simulink model "Ieee14_CC_2019b"  (R2019b)
settings: Solver=ode1  StartTime=0.0  StopTime=3600  FixedStep=1e-3  MaxStep=1e-4  RelTol=1e-3
model workspace (MAT data in the model file):
  pruebaValor = 0
libraries: powerlib x118, dspnetwork x112, source_mod x14, realtime_pacer_lib x1
(part 3 of 3)

== system Ieee14_CC_2019b/SM 5 ==
  Constant : Constant  Value=0
  Constant1 : Constant
  Constant2 : Constant  Value=2
  Constant3 : Constant  Value=0
  Constant4 : Constant
  Constant5 : Constant  Value=2
  Index Vector{,1..5} (6 alike) : MultiPortSwitch  DataPortOrder=Zero-based contiguous  Inputs=1  zeroidx=on
  Three-Phase V-I Measurement : powerlib/Measurements/Three-Phase V-I Measurement  VoltageMeasurement=phase-to-ground  SetLabelV=off  LabelV=Vabc  Vpu=on  VpuLL=off  CurrentMeasurement=yes  SetLabelI=off  LabelI=Iabc  Ipu=on  Pbase=100e6  Vbase=69e3  OutputType=Complex  PhasorSimulation=off  PSBequivalent=0
  UDP Send Ia : dspnetwork/UDP Send  remoteURL='10.0.255.255'  remotePort=20052  localURL='255.255.255.255'  localPortSource=Automatically determine  localPort=-1  sampletime=-1  blockPlatform=LINUX  separateLengthPort=0
  UDP Send Ib : dspnetwork/UDP Send  remoteURL='10.0.255.255'  remotePort=20051  localURL='255.255.255.255'  localPortSource=Automatically determine  localPort=-1  sampletime=-1  blockPlatform=LINUX  separateLengthPort=0
  UDP Send Ic : dspnetwork/UDP Send  remoteURL='10.0.255.255'  remotePort=20050  localURL='255.255.255.255'  localPortSource=Automatically determine  localPort=-1  sampletime=-1  blockPlatform=LINUX  separateLengthPort=0
  UDP Send Va : dspnetwork/UDP Send  remoteURL='10.0.255.255'  remotePort=10050  localURL='255.255.255.255'  localPortSource=Automatically determine  localPort=-1  sampletime=-1  blockPlatform=LINUX  separateLengthPort=0
  UDP Send Vb : dspnetwork/UDP Send  remoteURL='10.0.255.255'  remotePort=10051  localURL='255.255.255.255'  localPortSource=Automatically determine  localPort=-1  sampletime=-1  blockPlatform=LINUX  separateLengthPort=0
  UDP Send Vc : dspnetwork/UDP Send  remoteURL='10.0.255.255'  remotePort=10052  localURL='255.255.255.255'  localPortSource=Automatically determine  localPort=-1  sampletime=-1  blockPlatform=LINUX  separateLengthPort=0
  a : PMIOPort  Side=Left
  b : PMIOPort  Port=2  Side=Left
  c : PMIOPort  Port=3  Side=Left
  A : PMIOPort  Port=4  Side=Right
  B : PMIOPort  Port=5  Side=Right
  C : PMIOPort  Port=6  Side=Right
  Vabc : Outport
  Iabc : Outport  Port=2
  wires:
  Index Vector/1 -> UDP Send Va/1
  Constant1/1 -> Index Vector1/1
  Constant/1 -> Index Vector/1
  Index Vector2/1 -> UDP Send Vc/1
  Index Vector1/1 -> UDP Send Vb/1
  Constant2/1 -> Index Vector2/1
  Three-Phase V-I Measurement/1 -> Index Vector2/2, Index Vector/2, Index Vector1/2, Vabc/1
  Index Vector4/1 -> UDP Send Ib/1
  Constant3/1 -> Index Vector3/1
  Index Vector3/1 -> UDP Send Ic/1
  Constant5/1 -> Index Vector5/1
  Constant4/1 -> Index Vector4/1
  Index Vector5/1 -> UDP Send Ia/1
  Three-Phase V-I Measurement/2 -> Iabc/1, Index Vector3/2, Index Vector4/2, Index Vector5/2
  connections:
  b/RConn1 -- Three-Phase V-I Measurement/RConn2
  a/RConn1 -- Three-Phase V-I Measurement/RConn1
  c/RConn1 -- Three-Phase V-I Measurement/RConn3
  A/RConn1 -- Three-Phase V-I Measurement/LConn1
  B/RConn1 -- Three-Phase V-I Measurement/LConn2
  C/RConn1 -- Three-Phase V-I Measurement/LConn3

== system Ieee14_CC_2019b/SM 6 ==
  Constant : Constant  Value=0
  Constant1 : Constant
  Constant2 : Constant  Value=2
  Constant3 : Constant  Value=0
  Constant4 : Constant
  Constant5 : Constant  Value=2
  Index Vector{,1..5} (6 alike) : MultiPortSwitch  DataPortOrder=Zero-based contiguous  Inputs=1  zeroidx=on
  Three-Phase V-I Measurement : powerlib/Measurements/Three-Phase V-I Measurement  VoltageMeasurement=phase-to-ground  SetLabelV=off  LabelV=Vabc  Vpu=on  VpuLL=off  CurrentMeasurement=yes  SetLabelI=off  LabelI=Iabc  Ipu=on  Pbase=100e6  Vbase=69e3  OutputType=Complex  PhasorSimulation=off  PSBequivalent=0
  UDP Send Ia : dspnetwork/UDP Send  remoteURL='10.0.255.255'  remotePort=20062  localURL='255.255.255.255'  localPortSource=Automatically determine  localPort=-1  sampletime=-1  blockPlatform=LINUX  separateLengthPort=0
  UDP Send Ib : dspnetwork/UDP Send  remoteURL='10.0.255.255'  remotePort=20061  localURL='255.255.255.255'  localPortSource=Automatically determine  localPort=-1  sampletime=-1  blockPlatform=LINUX  separateLengthPort=0
  UDP Send Ic : dspnetwork/UDP Send  remoteURL='10.0.255.255'  remotePort=20060  localURL='255.255.255.255'  localPortSource=Automatically determine  localPort=-1  sampletime=-1  blockPlatform=LINUX  separateLengthPort=0
  UDP Send Va : dspnetwork/UDP Send  remoteURL='10.0.255.255'  remotePort=10060  localURL='255.255.255.255'  localPortSource=Automatically determine  localPort=-1  sampletime=-1  blockPlatform=LINUX  separateLengthPort=0
  UDP Send Vb : dspnetwork/UDP Send  remoteURL='10.0.255.255'  remotePort=10061  localURL='255.255.255.255'  localPortSource=Automatically determine  localPort=-1  sampletime=-1  blockPlatform=LINUX  separateLengthPort=0
  UDP Send Vc : dspnetwork/UDP Send  remoteURL='10.0.255.255'  remotePort=10062  localURL='255.255.255.255'  localPortSource=Automatically determine  localPort=-1  sampletime=-1  blockPlatform=LINUX  separateLengthPort=0
  a : PMIOPort  Side=Left
  b : PMIOPort  Port=2  Side=Left
  c : PMIOPort  Port=3  Side=Left
  A : PMIOPort  Port=4  Side=Right
  B : PMIOPort  Port=5  Side=Right
  C : PMIOPort  Port=6  Side=Right
  Vabc : Outport
  Iabc : Outport  Port=2
  wires:
  Index Vector/1 -> UDP Send Va/1
  Constant1/1 -> Index Vector1/1
  Constant/1 -> Index Vector/1
  Index Vector2/1 -> UDP Send Vc/1
  Index Vector1/1 -> UDP Send Vb/1
  Constant2/1 -> Index Vector2/1
  Three-Phase V-I Measurement/1 -> Index Vector2/2, Index Vector/2, Index Vector1/2, Vabc/1
  Index Vector4/1 -> UDP Send Ib/1
  Constant3/1 -> Index Vector3/1
  Index Vector3/1 -> UDP Send Ic/1
  Constant5/1 -> Index Vector5/1
  Constant4/1 -> Index Vector4/1
  Index Vector5/1 -> UDP Send Ia/1
  Three-Phase V-I Measurement/2 -> Iabc/1, Index Vector3/2, Index Vector4/2, Index Vector5/2
  connections:
  b/RConn1 -- Three-Phase V-I Measurement/RConn2
  a/RConn1 -- Three-Phase V-I Measurement/RConn1
  c/RConn1 -- Three-Phase V-I Measurement/RConn3
  A/RConn1 -- Three-Phase V-I Measurement/LConn1
  B/RConn1 -- Three-Phase V-I Measurement/LConn2
  C/RConn1 -- Three-Phase V-I Measurement/LConn3

== system Ieee14_CC_2019b/SM 7 ==
  Constant : Constant  Value=0
  Constant1 : Constant
  Constant2 : Constant  Value=2
  Constant3 : Constant  Value=0
  Constant4 : Constant
  Constant5 : Constant  Value=2
  Index Vector{,1..5} (6 alike) : MultiPortSwitch  DataPortOrder=Zero-based contiguous  Inputs=1  zeroidx=on
  Three-Phase V-I Measurement : powerlib/Measurements/Three-Phase V-I Measurement  VoltageMeasurement=phase-to-ground  SetLabelV=off  LabelV=Vabc  Vpu=on  VpuLL=off  CurrentMeasurement=yes  SetLabelI=off  LabelI=Iabc  Ipu=on  Pbase=100e6  Vbase=69e3  OutputType=Complex  PhasorSimulation=off  PSBequivalent=0
  UDP Send Ia : dspnetwork/UDP Send  remoteURL='10.0.255.255'  remotePort=20072  localURL='255.255.255.255'  localPortSource=Automatically determine  localPort=-1  sampletime=-1  blockPlatform=LINUX  separateLengthPort=0
  UDP Send Ib : dspnetwork/UDP Send  remoteURL='10.0.255.255'  remotePort=20071  localURL='255.255.255.255'  localPortSource=Automatically determine  localPort=-1  sampletime=-1  blockPlatform=LINUX  separateLengthPort=0
  UDP Send Ic : dspnetwork/UDP Send  remoteURL='10.0.255.255'  remotePort=20070  localURL='255.255.255.255'  localPortSource=Automatically determine  localPort=-1  sampletime=-1  blockPlatform=LINUX  separateLengthPort=0
  UDP Send Va : dspnetwork/UDP Send  remoteURL='10.0.255.255'  remotePort=10070  localURL='255.255.255.255'  localPortSource=Automatically determine  localPort=-1  sampletime=-1  blockPlatform=LINUX  separateLengthPort=0
  UDP Send Vb : dspnetwork/UDP Send  remoteURL='10.0.255.255'  remotePort=10071  localURL='255.255.255.255'  localPortSource=Automatically determine  localPort=-1  sampletime=-1  blockPlatform=LINUX  separateLengthPort=0
  UDP Send Vc : dspnetwork/UDP Send  remoteURL='10.0.255.255'  remotePort=10072  localURL='255.255.255.255'  localPortSource=Automatically determine  localPort=-1  sampletime=-1  blockPlatform=LINUX  separateLengthPort=0
  a : PMIOPort  Side=Left
  b : PMIOPort  Port=2  Side=Left
  c : PMIOPort  Port=3  Side=Left
  A : PMIOPort  Port=4  Side=Right
  B : PMIOPort  Port=5  Side=Right
  C : PMIOPort  Port=6  Side=Right
  Vabc : Outport
  Iabc : Outport  Port=2
  wires:
  Index Vector/1 -> UDP Send Va/1
  Constant1/1 -> Index Vector1/1
  Constant/1 -> Index Vector/1
  Index Vector2/1 -> UDP Send Vc/1
  Index Vector1/1 -> UDP Send Vb/1
  Constant2/1 -> Index Vector2/1
  Three-Phase V-I Measurement/1 -> Index Vector2/2, Index Vector/2, Index Vector1/2, Vabc/1
  Index Vector4/1 -> UDP Send Ib/1
  Constant3/1 -> Index Vector3/1
  Index Vector3/1 -> UDP Send Ic/1
  Constant5/1 -> Index Vector5/1
  Constant4/1 -> Index Vector4/1
  Index Vector5/1 -> UDP Send Ia/1
  Three-Phase V-I Measurement/2 -> Iabc/1, Index Vector3/2, Index Vector4/2, Index Vector5/2
  connections:
  b/RConn1 -- Three-Phase V-I Measurement/RConn2
  a/RConn1 -- Three-Phase V-I Measurement/RConn1
  c/RConn1 -- Three-Phase V-I Measurement/RConn3
  A/RConn1 -- Three-Phase V-I Measurement/LConn1
  B/RConn1 -- Three-Phase V-I Measurement/LConn2
  C/RConn1 -- Three-Phase V-I Measurement/LConn3

== system Ieee14_CC_2019b/SM 8 ==
  Constant : Constant  Value=0
  Constant1 : Constant
  Constant2 : Constant  Value=2
  Constant3 : Constant  Value=0
  Constant4 : Constant
  Constant5 : Constant  Value=2
  Index Vector{,1..5} (6 alike) : MultiPortSwitch  DataPortOrder=Zero-based contiguous  Inputs=1  zeroidx=on
  Three-Phase V-I Measurement : powerlib/Measurements/Three-Phase V-I Measurement  VoltageMeasurement=phase-to-ground  SetLabelV=off  LabelV=Vabc  Vpu=on  VpuLL=off  CurrentMeasurement=yes  SetLabelI=off  LabelI=Iabc  Ipu=on  Pbase=100e6  Vbase=69e3  OutputType=Complex  PhasorSimulation=off  PSBequivalent=0
  UDP Send Ia : dspnetwork/UDP Send  remoteURL='10.0.255.255'  remotePort=20082  localURL='255.255.255.255'  localPortSource=Automatically determine  localPort=-1  sampletime=-1  blockPlatform=LINUX  separateLengthPort=0
  UDP Send Ib : dspnetwork/UDP Send  remoteURL='10.0.255.255'  remotePort=20081  localURL='255.255.255.255'  localPortSource=Automatically determine  localPort=-1  sampletime=-1  blockPlatform=LINUX  separateLengthPort=0
  UDP Send Ic : dspnetwork/UDP Send  remoteURL='10.0.255.255'  remotePort=20080  localURL='255.255.255.255'  localPortSource=Automatically determine  localPort=-1  sampletime=-1  blockPlatform=LINUX  separateLengthPort=0
  UDP Send Va : dspnetwork/UDP Send  remoteURL='10.0.255.255'  remotePort=10080  localURL='255.255.255.255'  localPortSource=Automatically determine  localPort=-1  sampletime=-1  blockPlatform=LINUX  separateLengthPort=0
  UDP Send Vb : dspnetwork/UDP Send  remoteURL='10.0.255.255'  remotePort=10081  localURL='255.255.255.255'  localPortSource=Automatically determine  localPort=-1  sampletime=-1  blockPlatform=LINUX  separateLengthPort=0
  UDP Send Vc : dspnetwork/UDP Send  remoteURL='10.0.255.255'  remotePort=10082  localURL='255.255.255.255'  localPortSource=Automatically determine  localPort=-1  sampletime=-1  blockPlatform=LINUX  separateLengthPort=0
  a : PMIOPort  Side=Left
  b : PMIOPort  Port=2  Side=Left
  c : PMIOPort  Port=3  Side=Left
  A : PMIOPort  Port=4  Side=Right
  B : PMIOPort  Port=5  Side=Right
  C : PMIOPort  Port=6  Side=Right
  Vabc : Outport
  Iabc : Outport  Port=2
  wires:
  Index Vector/1 -> UDP Send Va/1
  Constant1/1 -> Index Vector1/1
  Constant/1 -> Index Vector/1
  Index Vector2/1 -> UDP Send Vc/1
  Index Vector1/1 -> UDP Send Vb/1
  Constant2/1 -> Index Vector2/1
  Three-Phase V-I Measurement/1 -> Index Vector2/2, Index Vector/2, Index Vector1/2, Vabc/1
  Index Vector4/1 -> UDP Send Ib/1
  Constant3/1 -> Index Vector3/1
  Index Vector3/1 -> UDP Send Ic/1
  Constant5/1 -> Index Vector5/1
  Constant4/1 -> Index Vector4/1
  Index Vector5/1 -> UDP Send Ia/1
  Three-Phase V-I Measurement/2 -> Iabc/1, Index Vector3/2, Index Vector4/2, Index Vector5/2
  connections:
  b/RConn1 -- Three-Phase V-I Measurement/RConn2
  a/RConn1 -- Three-Phase V-I Measurement/RConn1
  c/RConn1 -- Three-Phase V-I Measurement/RConn3
  A/RConn1 -- Three-Phase V-I Measurement/LConn1
  B/RConn1 -- Three-Phase V-I Measurement/LConn2
  C/RConn1 -- Three-Phase V-I Measurement/LConn3

== system Ieee14_CC_2019b/SM 9 ==
  Constant : Constant  Value=0
  Constant1 : Constant
  Constant2 : Constant  Value=2
  Constant3 : Constant  Value=0
  Constant4 : Constant
  Constant5 : Constant  Value=2
  Index Vector{,1..5} (6 alike) : MultiPortSwitch  DataPortOrder=Zero-based contiguous  Inputs=1  zeroidx=on
  Three-Phase V-I Measurement : powerlib/Measurements/Three-Phase V-I Measurement  VoltageMeasurement=phase-to-ground  SetLabelV=off  LabelV=Vabc  Vpu=on  VpuLL=off  CurrentMeasurement=yes  SetLabelI=off  LabelI=Iabc  Ipu=on  Pbase=100e6  Vbase=69e3  OutputType=Complex  PhasorSimulation=off  PSBequivalent=0
  UDP Send Ia : dspnetwork/UDP Send  remoteURL='10.0.255.255'  remotePort=20092  localURL='255.255.255.255'  localPortSource=Automatically determine  localPort=-1  sampletime=-1  blockPlatform=LINUX  separateLengthPort=0
  UDP Send Ib : dspnetwork/UDP Send  remoteURL='10.0.255.255'  remotePort=20091  localURL='255.255.255.255'  localPortSource=Automatically determine  localPort=-1  sampletime=-1  blockPlatform=LINUX  separateLengthPort=0
  UDP Send Ic : dspnetwork/UDP Send  remoteURL='10.0.255.255'  remotePort=20090  localURL='255.255.255.255'  localPortSource=Automatically determine  localPort=-1  sampletime=-1  blockPlatform=LINUX  separateLengthPort=0
  UDP Send Va : dspnetwork/UDP Send  remoteURL='10.0.255.255'  remotePort=10090  localURL='255.255.255.255'  localPortSource=Automatically determine  localPort=-1  sampletime=-1  blockPlatform=LINUX  separateLengthPort=0
  UDP Send Vb : dspnetwork/UDP Send  remoteURL='10.0.255.255'  remotePort=10091  localURL='255.255.255.255'  localPortSource=Automatically determine  localPort=-1  sampletime=-1  blockPlatform=LINUX  separateLengthPort=0
  UDP Send Vc : dspnetwork/UDP Send  remoteURL='10.0.255.255'  remotePort=10092  localURL='255.255.255.255'  localPortSource=Automatically determine  localPort=-1  sampletime=-1  blockPlatform=LINUX  separateLengthPort=0
  a : PMIOPort  Side=Left
  b : PMIOPort  Port=2  Side=Left
  c : PMIOPort  Port=3  Side=Left
  A : PMIOPort  Port=4  Side=Right
  B : PMIOPort  Port=5  Side=Right
  C : PMIOPort  Port=6  Side=Right
  Vabc : Outport
  Iabc : Outport  Port=2
  wires:
  Index Vector/1 -> UDP Send Va/1
  Constant1/1 -> Index Vector1/1
  Constant/1 -> Index Vector/1
  Index Vector2/1 -> UDP Send Vc/1
  Index Vector1/1 -> UDP Send Vb/1
  Constant2/1 -> Index Vector2/1
  Three-Phase V-I Measurement/1 -> Index Vector2/2, Index Vector/2, Index Vector1/2, Vabc/1
  Index Vector4/1 -> UDP Send Ib/1
  Constant3/1 -> Index Vector3/1
  Index Vector3/1 -> UDP Send Ic/1
  Constant5/1 -> Index Vector5/1
  Constant4/1 -> Index Vector4/1
  Index Vector5/1 -> UDP Send Ia/1
  Three-Phase V-I Measurement/2 -> Iabc/1, Index Vector3/2, Index Vector4/2, Index Vector5/2
  connections:
  b/RConn1 -- Three-Phase V-I Measurement/RConn2
  a/RConn1 -- Three-Phase V-I Measurement/RConn1
  c/RConn1 -- Three-Phase V-I Measurement/RConn3
  A/RConn1 -- Three-Phase V-I Measurement/LConn1
  B/RConn1 -- Three-Phase V-I Measurement/LConn2
  C/RConn1 -- Three-Phase V-I Measurement/LConn3

== matlab function Ieee14_CC_2019b/CC ==
  settings: updateMethod=DISCRETE  sampleTime=10
function fcn()

    %{
    
    Function CC: short circuits.
    
    Details: This function is responsible for causing short circuits throughout the simulation.
    
    Important: In edit Data, you must adjust the time interval for entering this function. If the interval is set to 5 seconds, its behavior is:
    
    T = 5s --> A random fault is activated
    T = 10s --> The fault is deactivated
    T = 15s --> A random fault is activated
    T = 20s --> The fault is deactivated
    ... ... ...
    
    %}

    
    % - - - - - - - - - - - - - - - - - - - - - - - - -
    
    % coders
    coder.extrinsic('mat2str');
    coder.extrinsic('set_param');
    
    % - - - - - - - - - - - - - - - - - - - - - - - - -
    
    % If skip=1, no fault is activated
    skip = 0;
    
    % - - - - - - - - - - - - - - - - - - - - - - - - -
    
    % = = = = = = = = = = = = = = = = = = = = = = = = =
    % = = = = = = = = = = = = = = = = = = = = = = = = =
    % - - - - - - - - Code - - - - - - - - - - - - - 
    % = = = = = = = = = = = = = = = = = = = = = = = = =
    % = = = = = = = = = = = = = = = = = = = = = = = = =
    
    % - - - - - - - - - - - - - - - - - - - - - - - - -
    
    % Activate or skip fault generation
    if skip == 1
        return
    end
    
    % - - - - - - - - - - - - - - - - - - - - - - - - -
    
    % Persisten variables
    
    % attack: if 1, fault is activated (cc)
    persistent fault_active
    if isempty(fault_active)
       fault_active = 0;
       return
    end
    
    % lineCC: line with active fault
    persistent lineCC;
    if isempty(lineCC)
        lineCC = 0;
    end
    
    % - - - - - - - - - - - - - - - - - - - - - - - - -
    
    % Model path
    path = "Ieee14_CC/";
    
    % - - - - - - - - - - - - - - - - - - - - - - - - -
    
    % Restore ataque
    if fault_active == 1
        if lineCC == 0
            line = "L0";
            aux = path + "CC_" + line;
            set_param(aux, 'Value', mat2str(0));
        end
        if lineCC == 1
            line = "L1";
            aux = path + "CC_" + line;
            set_param(aux, 'Value', mat2str(0));
        end
        if lineCC == 2
            line = "L2";
            aux = path + "CC_" + line;
            set_param(aux, 'Value', mat2str(0));
        end
        if lineCC == 3
            line = "L3";
            aux = path + "CC_" + line;
            set_param(aux, 'Value', mat2str(0));
        end
        if lineCC == 4
            line = "L4";
            aux = path + "CC_" + line;
            set_param(aux, 'Value', mat2str(0));
        end
        if lineCC == 5
            line = "L5";
            aux = path + "CC_" + line;
            set_param(aux, 'Value', mat2str(0));
        end
        if lineCC == 6
            line = "L6";
            aux = path + "CC_" + line;
            set_param(aux, 'Value', mat2str(0));
        end
        if lineCC == 7
            line = "L7";
            aux = path + "CC_" + line;
            set_param(aux, 'Value', mat2str(0));
        end
        if lineCC == 8
            line = "L8";
            aux = path + "CC_" + line;
            set_param(aux, 'Value', mat2str(0));
        end
        if lineCC == 9
            line = "L9";
            aux = path + "CC_" + line;
            set_param(aux, 'Value', mat2str(0));
        end
        if lineCC == 10
            line = "L10";
            aux = path + "CC_" + line;
            set_param(aux, 'Value', mat2str(0));
        end
        if lineCC == 11
            line = "L11";
            aux = path + "CC_" + line;
            set_param(aux, 'Value', mat2str(0));
        end
        if lineCC == 12
            line = "L12";
            aux = path + "CC_" + line;
            set_param(aux, 'Value', mat2str(0));
        end
        if lineCC == 13
            line = "L13";
            aux = path + "CC_" + line;
            set_param(aux, 'Value', mat2str(0));
        end
        if lineCC == 14
            line = "L14";
            aux = path + "CC_" + line;
            set_param(aux, 'Value', mat2str(0));
        end
        if lineCC == 15
            line = "L15";
            aux = path + "CC_" + line;
            set_param(aux, 'Value', mat2str(0));
        end
    
        fault_active = 0;
        disp('=============')
        disp('Disconnection CC');
        disp('=============');
        return
    end
    
    % Activate fault

    % Probability of 10% of line failing
    activate = randi(10);
    
    if fault_active == 0 && activate
        % Randomly select line (0-15)
        lineCC = randi(16) - 1;
        disp('=======================');
        disp('=======================');
        disp('LineaCC');
        disp(lineCC);
        disp('=======================');
        disp('=======================');
        if lineCC == 0
            line = "L0";
            aux = path + "CC_" + line;
            set_param(aux, 'Value', mat2str(1));
        end
        if lineCC == 1
            line = "L1";
            aux = path + "CC_" + line;
            set_param(aux, 'Value', mat2str(1));
        end
        if lineCC == 2
            line = "L2";
            aux = path + "CC_" + line;
            set_param(aux, 'Value', mat2str(1));
        end
        if lineCC == 3
            line = "L3";
            aux = path + "CC_" + line;
            set_param(aux, 'Value', mat2str(1));
        end
        if lineCC == 4
            line = "L4";
            aux = path + "CC_" + line;
            set_param(aux, 'Value', mat2str(1));
        end
        if lineCC == 5
            line = "L5";
            aux = path + "CC_" + line;
            set_param(aux, 'Value', mat2str(1));
        end
        if lineCC == 6
            line = "L6";
            aux = path + "CC_" + line;
            set_param(aux, 'Value', mat2str(1));
        end
        if lineCC == 7
            line = "L7";
            aux = path + "CC_" + line;
            set_param(aux, 'Value', mat2str(1));
        end
        if lineCC == 8
            line = "L8";
            aux = path + "CC_" + line;
            set_param(aux, 'Value', mat2str(1));
        end
        if lineCC == 9
            line = "L9";
            aux = path + "CC_" + line;
            set_param(aux, 'Value', mat2str(1));
        end
        if lineCC == 10
            line = "L10";
            aux = path + "CC_" + line;
            set_param(aux, 'Value', mat2str(1));
        end
        if lineCC == 11
            line = "L11";
            aux = path + "CC_" + line;
            set_param(aux, 'Value', mat2str(1));
        end
        if lineCC == 12
            line = "L12";
            aux = path + "CC_" + line;
            set_param(aux, 'Value', mat2str(1));
        end
        if lineCC == 13
            line = "L13";
            aux = path + "CC_" + line;
            set_param(aux, 'Value', mat2str(1));
        end
        if lineCC == 14
            line = "L14";
            aux = path + "CC_" + line;
            set_param(aux, 'Value', mat2str(1));
        end
        if lineCC == 15
            line = "L15";
            aux = path + "CC_" + line;
            set_param(aux, 'Value', mat2str(1));
        end
        fault_active = 1;
        return
    end

end

== matlab function Ieee14_CC_2019b/InicioFcn ==
  settings: sampleTime=0
  data: u input
function fcn(u)

%{

Funcion: inicioFcn

Detalles: Funcion de inicializacion de la red. Se ejecuta 1 sola vez. 
Llama a la funcion resetRed externa que inicializa los valores de la red.

Adicional: Para evitar cualquier mensaje de warning, se anulan desde la
linea warning('off','all'). A pesar del warning, no es un problema para el
funcionamiento de la red

%}

% - - - - - - - - - - - - - - - - - - - - - - - - -

% Coder
coder.extrinsic('resetRed');
coder.extrinsic('warning');

% - - - - - - - - - - - - - - - - - - - - - - - - -

% Resetar
if u == 0
    resetRed();
    warning('off','all');
end

% - - - - - - - - - - - - - - - - - - - - - - - - -
end
